simulink model "Signal_Mixer"  (R2022a)
settings: Solver=FixedStepAuto  StartTime=0.0  StopTime=10  FixedStep=1/Fs  RelTol=1e-3
values from neighbouring files (symbols this model uses):
  alpha_AC = 1    [basic.m]    (also in test.m = 0.7)
  alpha_AD = 1    [basic.m]    (also in test.m = 0.3)
  alpha_BC = 1    [basic.m]    (also in test.m = 0.2)
  alpha_BD = 1    [basic.m]    (also in test.m = 0.8)
  beta_AC = floor(.002*Fs)    [basic.m]    (also in test.m = floor(.1*Fs))
  beta_AD = floor(.001*Fs)    [basic.m]    (also in test.m = floor(.3*Fs))
  beta_BC = floor(.002*Fs)    [basic.m]    (also in test.m = floor(.7*Fs))
  beta_BD = floor(.004*Fs)    [basic.m]    (also in test.m = floor(.01*Fs))
settings Model: Creator=yash2  LastModifiedBy=Yash
settings DebuggingCC: UnconnectedInputMsg=warning  UnconnectedOutputMsg=warning  UnconnectedLineMsg=warning
settings RTWCC: DLArmComputeVersion=19.05

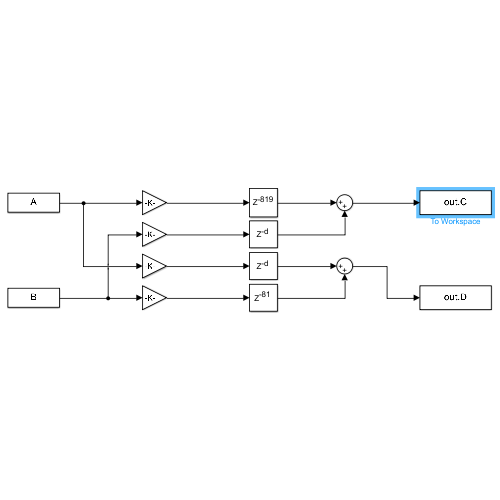
[thumbnail: Simulink's stored preview of the top-level diagram]
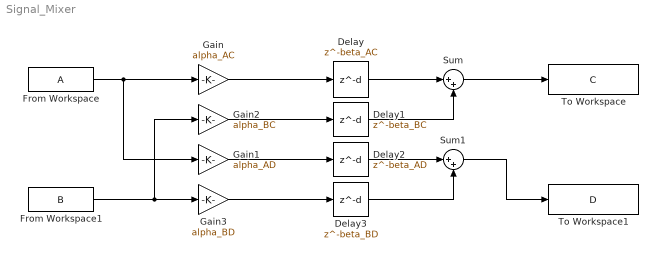
== system Signal_Mixer ==
  Delay : Delay  DelayLength=beta_AC  InitialCondition=0
  Delay1 : Delay  DelayLength=beta_BC  InitialCondition=0
  Delay2 : Delay  DelayLength=beta_AD  InitialCondition=0
  Delay3 : Delay  DelayLength=beta_BD  InitialCondition=0
  From Workspace : FromWorkspace  VariableName=A  OutputAfterFinalValue=Setting to zero
  From Workspace1 : FromWorkspace  VariableName=B  OutputAfterFinalValue=Setting to zero
  Gain : Gain  Gain=alpha_AC
  Gain1 : Gain  Gain=alpha_AD
  Gain2 : Gain  Gain=alpha_BC
  Gain3 : Gain  Gain=alpha_BD
  Sum : Sum  Inputs=|++
  Sum1 : Sum  Inputs=|++
  To Workspace : ToWorkspace  VariableName=C  SaveFormat=Timeseries  SampleTime=-1
      settings: Save2DSignal=2-D array (concatenate along first dimension)
  To Workspace1 : ToWorkspace  VariableName=D  SaveFormat=Timeseries  SampleTime=-1
      settings: Save2DSignal=2-D array (concatenate along first dimension)
  wires:
  Gain1/1 -> Delay2/1
  Gain3/1 -> Delay3/1
  Gain/1 -> Delay/1
  Delay3/1 -> Sum1/2
  From Workspace1/1 -> Gain2/1, Gain3/1
  Delay2/1 -> Sum1/1
  Delay1/1 -> Sum/2
  Gain2/1 -> Delay1/1
  Delay/1 -> Sum/1
  From Workspace/1 -> Gain/1, Gain1/1
  Sum1/1 -> To Workspace1/1
  Sum/1 -> To Workspace/1
